simulink library "collection_of_goodies"  (R2018a)
settings: Solver=VariableStepAuto  StartTime=0.0  StopTime=10.0  RelTol=1e-3
undefined symbols (not defined in the file or in its folder): a1_T_CMG, a2_T_CMG, a3_T_CMG, AccLim, b1_T_CMG, b2_T_CMG, b3_T_CMG, c, CFthreshoff, CFthreshon, filt1d, filt1n, filt2d, filt2n, filts1n, filts2d, filts2n, fine, h, h_cos_cmg, h_init, h_sin_cmg, hdmax, hmax, I, I34, Id, Igm1d, Igm1n, IgmAAFd, init, invI, invId, Is, Isat, IsatSp, k1_obs, k2_obs, Kt, Kts, lam, Lgm, ls, lt, M34, Ngear, P0, pfd, pfn, q0, q_init, rc_ampl, rc_harm, rc_phase, Rgm, Smin, SmotDrag, spin_init, TachAAFd, TAU_ACS ... (+9)
libraries: mblibv1 x3, sharedutil x1, dspinverses x1, $bdroot x1
(part 3 of 3)

== system collection_of_goodies/Attitude Dynamics/CMG Gimbal Control System/Sensor/Tach Phases ==
  note: Add model of each phase based on truth angle,
      | then mux to one per Tach Commutation input
  TachComm : Inport
  Rate : Inport  Port=2
  Truth Angle : Inport  Port=3
  Meas Rate : Outport  InitialOutput=0
  wires:
  Rate/1 -> Meas Rate/1

== system collection_of_goodies/Attitude Dynamics/CMG Gimbal Control System/Sensor/Tach Ripple ==
  note: Ripple
      | Factor
  note: Ripple
      | Term
  Rate In : Inport
  Motor Angle : Inport  Port=2
  Amplitude : Constant  Value=tr_ampl
  Demux : Demux  Outputs=[2 8]
  Harmonic : Constant  Value=tr_harm
  Phase : Constant  Value=tr_phase
  Product : Product  SaturateOnIntegerOverflow=on  InputSameDT=on  OutDataTypeStr=Inherit: Same as first input
  Product1 : Product  SaturateOnIntegerOverflow=on  InputSameDT=on  OutDataTypeStr=Inherit: Same as first input
  Product2 : Product  SaturateOnIntegerOverflow=on  InputSameDT=on  OutDataTypeStr=Inherit: Same as first input
  Sum : Sum  Inputs=++|  SaturateOnIntegerOverflow=on  InputSameDT=on  OutDataTypeStr=Inherit: Same as first input
  Sum3 : Sum  Inputs=+  SaturateOnIntegerOverflow=on  InputSameDT=on  OutDataTypeStr=Inherit: Same as first input
  Sum4 : Sum  Inputs=+  SaturateOnIntegerOverflow=on  InputSameDT=on  OutDataTypeStr=Inherit: Same as first input
  Sum5 : Sum  SaturateOnIntegerOverflow=on  InputSameDT=on  OutDataTypeStr=Inherit: Same as first input
  Trigonometric Function : Trigonometry  Operator=cos
  Tach Ripple : Outport  InitialOutput=0
  wires:
  Sum5/1 -> Tach Ripple/1
  Product1/1 -> Sum5/2
  Demux/2 -> Sum4/1
  Demux/1 -> Sum3/1
  Amplitude/1 -> Product2/2
  Harmonic/1 -> Product/2
  Product2/1 -> Demux/1
  Trigonometric Function/1 -> Product2/1
  Product/1 -> Trigonometric Function/1
  Rate In/1 -> Product1/2
  Sum4/1 -> Product1/1
  Sum3/1 -> Sum5/1
  Phase/1 -> Sum/1
  Motor Angle/1 -> Sum/2
  Sum/1 -> Product/1

== system collection_of_goodies/Attitude Dynamics/Rigid Body with Momentum Actuators and energy dissipation/Quaternion Integration/q_normalize ==
  q_in : Inport  PortDimensions=4
  Dot Product : DotProduct  InputSameDT=on  OutDataTypeStr=Inherit: Inherit via internal rule
  Math Function : Math  Operator=sqrt  SaturateOnIntegerOverflow=on
  Product : Product  Inputs=*/  SaturateOnIntegerOverflow=on  InputSameDT=on  OutDataTypeStr=Inherit: Same as first input
  q_out : Outport
  wires:
  q_in/1 -> Dot Product/1, Dot Product/2, Product/1
  Dot Product/1 -> Math Function/1
  Math Function/1 -> Product/2
  Product/1 -> q_out/1

== system collection_of_goodies/Attitude Dynamics/Rigid Body with Momentum Actuators and energy dissipation/Quaternion Integration/qderiv ==
  w : Inport
  q : Inport  Port=2
  Mux : Mux  Inputs=2
  Mux1 : Mux
  qd1 : Fcn  Expr=(u(7)*u(1)-u(6)*u(2)+u(5)*u(3))/2
  qd2 : Fcn  Expr=(u(6)*u(1)+u(7)*u(2)-u(4)*u(3))/2
  qd3 : Fcn  Expr=(-u(5)*u(1)+u(4)*u(2)+u(7)*u(3))/2
  qd4 : Fcn  Expr=(-u(4)*u(1)-u(5)*u(2)-u(6)*u(3))/2
  qd : Outport
  wires:
  w/1 -> Mux/1
  q/1 -> Mux/2
  Mux/1 -> qd1/1, qd2/1, qd3/1, qd4/1
  qd1/1 -> Mux1/1
  qd2/1 -> Mux1/2
  qd3/1 -> Mux1/3
  qd4/1 -> Mux1/4
  Mux1/1 -> qd/1

== matlab function collection_of_goodies/Environment/Reference Sun Kepler/MATLAB Function ==
  data: t input; S output; tp input; yearT input; e input; q input
function S = fcn(t,tp,yearT,e,q)
%sds
S= refSunK(t,tp,yearT,e,q);
